simulink model "scara_2018a"  (R2018a)
settings: Solver=VariableStepAuto  StartTime=0.0  StopTime=inf  RelTol=1e-3
libraries: simulink x4, simulink_extras x2
settings Model: Creator=Bartlomiej Mroz  LastModifiedBy=Duch Kraftu
settings DebuggingCC: LibraryContextMissingDiagnostic=warning
settings SFSimCC: SimUseLocalCustomCode=on
settings RTWCC: RTWUseLocalCustomCode=on

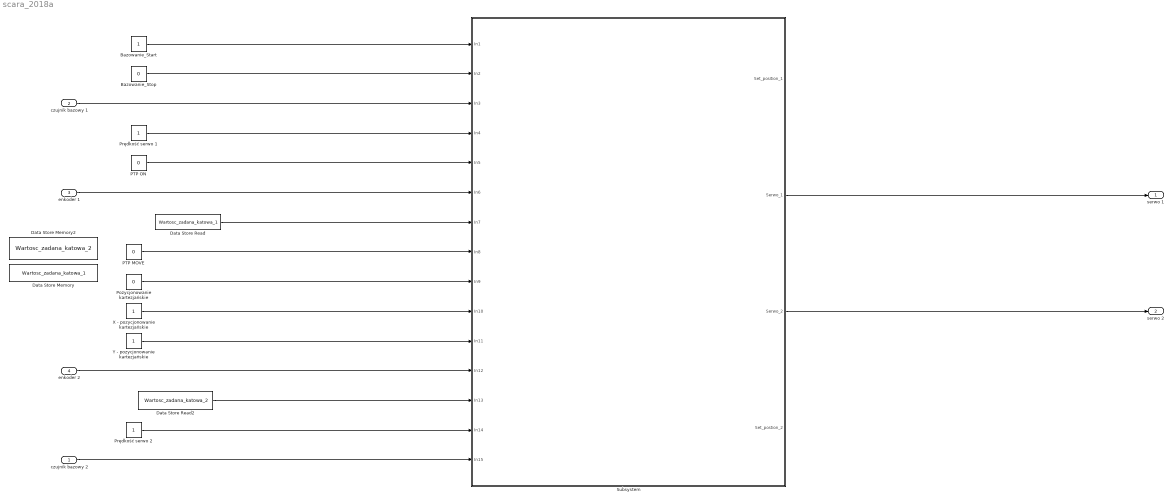
== system scara_2018a ==
  czujnik bazowy 2 : Inport
  czujnik bazowy 1 : Inport  Port=2
  enkoder 1 : Inport  Port=3
  enkoder 2 : Inport  Port=4
  " Bazowanie_Stop" : Constant  Value=0
  Bazowanie_Start : Constant
  Data Store Memory : DataStoreMemory  DataStoreName=Wartosc_zadana_katowa_1  ReadBeforeWriteMsg=warning  WriteAfterWriteMsg=warning  WriteAfterReadMsg=warning  ShowAdditionalParam=off
  Data Store Memory2 : DataStoreMemory  DataStoreName=Wartosc_zadana_katowa_2  ReadBeforeWriteMsg=warning  WriteAfterWriteMsg=warning  WriteAfterReadMsg=warning  ShowAdditionalParam=off
  Data Store Read : DataStoreRead  DataStoreName=Wartosc_zadana_katowa_1
  Data Store Read2 : DataStoreRead  DataStoreName=Wartosc_zadana_katowa_2
  PTP MOVE : Constant  Value=0
  "PTP ON " : Constant  Value=0
  "Pozycjonowanie kartezjańskie " : Constant  Value=0
  Prędkość serwo 1 : Constant
  Prędkość serwo 2 : Constant
  Subsystem : Subsystem
  X - pozycjonowanie kartezjańskie : Constant
  Y - pozycjonowanie kartezjańskie : Constant
  serwo 1 : Outport  VectorParamsAs1DForOutWhenUnconnected=on
  serwo 2 : Outport  Port=2  VectorParamsAs1DForOutWhenUnconnected=on
  wires:
  Bazowanie_Start/1 -> Subsystem/1(In1)
  " Bazowanie_Stop"/1 -> Subsystem/2(In2)
  czujnik bazowy 1/1 -> Subsystem/3(In3)
  Prędkość serwo 1/1 -> Subsystem/4(In4)
  "PTP ON "/1 -> Subsystem/5(In5)
  enkoder 1/1 -> Subsystem/6(In6)
  Data Store Read/1 -> Subsystem/7(In7)
  PTP MOVE/1 -> Subsystem/8(In8)
  "Pozycjonowanie kartezjańskie "/1 -> Subsystem/9(In9)
  X - pozycjonowanie kartezjańskie/1 -> Subsystem/10(In10)
  Y - pozycjonowanie kartezjańskie/1 -> Subsystem/11(In11)
  enkoder 2/1 -> Subsystem/12(In12)
  Data Store Read2/1 -> Subsystem/13(In13)
  Prędkość serwo 2/1 -> Subsystem/14(In14)
  czujnik bazowy 2/1 -> Subsystem/15(In15)
  Subsystem/2(Serwo_1) -> serwo 1/1
  Subsystem/3(Serwo_2) -> serwo 2/1

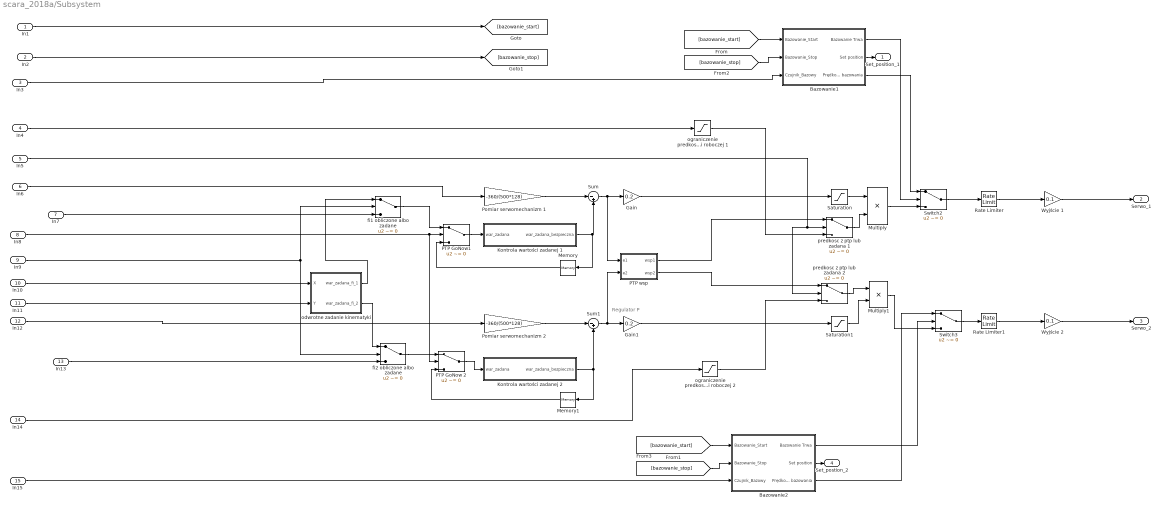
== system scara_2018a/Subsystem ==
  note: Regulator P
  In1 : Inport
  In2 : Inport  Port=2
  In3 : Inport  Port=3
  In4 : Inport  Port=4
  In5 : Inport  Port=5
  In6 : Inport  Port=6
  In7 : Inport  Port=7
  In8 : Inport  Port=8
  In9 : Inport  Port=9
  In10 : Inport  Port=10
  In11 : Inport  Port=11
  In12 : Inport  Port=12
  In13 : Inport  Port=13
  In14 : Inport  Port=14
  In15 : Inport  Port=15
  Bazowanie1 : Subsystem
  Bazowanie2 : Subsystem
  Gain : Gain  Gain=0.2
  Gain1 : Gain  Gain=0.2
  "Kontrola wartości zadanej 1 " : Subsystem
  Kontrola wartości zadanej 2 : Subsystem
  Memory : Memory
  Memory1 : Memory
  Multiply : Product
  Multiply1 : Product
  PTP GoNow 2 : Switch  Criteria=u2 ~= 0
  PTP GoNow1 : Switch  Criteria=u2 ~= 0
  "PTP wsp " : MATLAB Function  TreatAsAtomicUnit=on
  Pomiar serwomechanizm 1 : Gain  Gain=-360/(500*128)
  Pomiar serwomechanizm 2 : Gain  Gain=-360/(500*128)
  Rate Limiter : RateLimiter  RisingSlewLimit=50  FallingSlewLimit=-50  SampleTimeMode=inherited
  Rate Limiter1 : RateLimiter  RisingSlewLimit=50  FallingSlewLimit=-50  SampleTimeMode=inherited
  Saturation : Saturate  UpperLimit=3  LowerLimit=-3
  Saturation1 : Saturate  UpperLimit=3  LowerLimit=-3
  Sum : Sum  Inputs=|-+
  Sum1 : Sum  Inputs=|-+
  Switch2 : Switch  Criteria=u2 ~= 0
  Switch3 : Switch  Criteria=u2 ~= 0
  Wyjście 1 : Gain  Gain=0.1
  Wyjście 2 : Gain  Gain=0.1
  fi1 obliczone albo zadane : Switch  Criteria=u2 ~= 0
  fi2 obliczone albo zadane : Switch  Criteria=u2 ~= 0
  odwrotne zadanie kinematyki : Subsystem
  ograniczenie predkosci roboczej 1 : Saturate  UpperLimit=1  LowerLimit=0.05
  ograniczenie predkosci roboczej 2 : Saturate  UpperLimit=1  LowerLimit=0.05
  predkosc z ptp lub zadana 1 : Switch  Criteria=u2 ~= 0
  predkosc z ptp lub zadana 2 : Switch  Criteria=u2 ~= 0
  Set_position_1 : Outport  VectorParamsAs1DForOutWhenUnconnected=on
  Serwo_1 : Outport  Port=2  VectorParamsAs1DForOutWhenUnconnected=on
  Serwo_2 : Outport  Port=3  VectorParamsAs1DForOutWhenUnconnected=on
  Set_postion_2 : Outport  Port=4  VectorParamsAs1DForOutWhenUnconnected=on
  wires:
  In8/1 -> PTP GoNow 2/2, PTP GoNow1/2
  Bazowanie1/3(Prędkość bazowania) -> Switch2/1
  [bazowanie_start] -> Bazowanie1/1(Bazowanie_Start)
  Kontrola wartości zadanej 2/1(war_zadana_bezpieczna) -> Memory1/1, Sum1/2
  [bazowanie_stop] -> Bazowanie1/2("Bazowanie_Stop ")
  In9/1 -> fi1 obliczone albo zadane/2, fi2 obliczone albo zadane/2
  Bazowanie1/1("Bazowanie Trwa ") -> Switch2/2
  Multiply/1 -> Switch2/3
  Gain1/1 -> Saturation1/1
  [bazowanie_start] -> Bazowanie2/1(Bazowanie_Start)
  Sum/1 -> Gain/1, "PTP wsp "/1(e1)
  predkosc z ptp lub zadana 2/1 -> Multiply1/1
  [bazowanie_stop] -> Bazowanie2/2("Bazowanie_Stop ")
  In15/1 -> Bazowanie2/3(Czujnik_Bazowy)
  In12/1 -> Pomiar serwomechanizm 2/1
  ograniczenie predkosci roboczej 1/1 -> predkosc z ptp lub zadana 1/3
  Gain/1 -> Saturation/1
  ograniczenie predkosci roboczej 2/1 -> predkosc z ptp lub zadana 2/3
  In3/1 -> Bazowanie1/3(Czujnik_Bazowy)
  "Kontrola wartości zadanej 1 "/1(war_zadana_bezpieczna) -> Memory/1, Sum/2
  Bazowanie2/2("Set position ") -> Set_postion_2/1
  Sum1/1 -> Gain1/1, "PTP wsp "/2(e2)
  In5/1 -> predkosc z ptp lub zadana 2/2, predkosc z ptp lub zadana 1/2
  fi1 obliczone albo zadane/1 -> PTP GoNow1/1
  Saturation/1 -> Multiply/1
  Memory1/1 -> PTP GoNow 2/3
  Rate Limiter1/1 -> Wyjście 2/1
  Pomiar serwomechanizm 1/1 -> Sum/1
  Saturation1/1 -> Multiply1/2
  In6/1 -> Pomiar serwomechanizm 1/1
  In4/1 -> ograniczenie predkosci roboczej 1/1
  "PTP wsp "/2(wsp2) -> predkosc z ptp lub zadana 2/1
  Wyjście 1/1 -> Serwo_1/1
  In11/1 -> odwrotne zadanie kinematyki/2(Y)
  Pomiar serwomechanizm 2/1 -> Sum1/1
  fi2 obliczone albo zadane/1 -> PTP GoNow 2/1
  Wyjście 2/1 -> Serwo_2/1
  Bazowanie2/3(Prędkość bazowania) -> Switch3/1
  PTP GoNow 2/1 -> Kontrola wartości zadanej 2/1(war_zadana)
  odwrotne zadanie kinematyki/2(war_zadana_fi_2) -> fi2 obliczone albo zadane/1
  Switch3/1 -> Rate Limiter1/1
  Bazowanie2/1("Bazowanie Trwa ") -> Switch3/2
  PTP GoNow1/1 -> "Kontrola wartości zadanej 1 "/1(war_zadana)
  Memory/1 -> PTP GoNow1/3
  In14/1 -> ograniczenie predkosci roboczej 2/1
  predkosc z ptp lub zadana 1/1 -> Multiply/2
  Rate Limiter/1 -> Wyjście 1/1
  Switch2/1 -> Rate Limiter/1
  odwrotne zadanie kinematyki/1(war_zadana_fi_1) -> fi1 obliczone albo zadane/1
  In2/1 -> [bazowanie_stop]
  Multiply1/1 -> Switch3/3
  "PTP wsp "/1(wsp1) -> predkosc z ptp lub zadana 1/1
  In1/1 -> [bazowanie_start]
  In7/1 -> fi1 obliczone albo zadane/3
  Bazowanie1/2("Set position ") -> Set_position_1/1
  In13/1 -> fi2 obliczone albo zadane/3
  In10/1 -> odwrotne zadanie kinematyki/1(X)

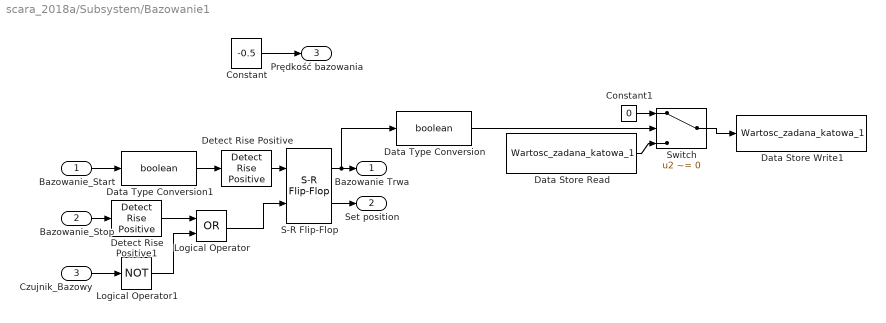
== system scara_2018a/Subsystem/Bazowanie1 ==
  Bazowanie_Start : Inport
  "Bazowanie_Stop " : Inport  Port=2
  Czujnik_Bazowy : Inport  Port=3
  Constant : Constant  Value=-0.5
  Constant1 : Constant  Value=0
  Data Store Read : DataStoreRead  DataStoreName=Wartosc_zadana_katowa_1
  Data Store Write1 : DataStoreWrite  DataStoreName=Wartosc_zadana_katowa_1
  Data Type Conversion : DataTypeConversion  OutDataTypeStr=boolean
  Data Type Conversion1 : DataTypeConversion  OutDataTypeStr=boolean
  Detect Rise Positive : simulink/Logic and Bit Operations/Detect Rise Positive  vinit=0  OutDataTypeStr=boolean
  Detect Rise Positive1 : simulink/Logic and Bit Operations/Detect Rise Positive  vinit=0  OutDataTypeStr=boolean
  Logical Operator : Logic  Operator=OR  AllPortsSameDT=off  OutDataTypeStr=boolean
  Logical Operator1 : Logic  Operator=NOT  AllPortsSameDT=off  OutDataTypeStr=boolean
  S-R Flip-Flop : simulink_extras/Flip Flops/S-R Flip-Flop  initial_condition=0
  Switch : Switch  Criteria=u2 ~= 0
  "Bazowanie Trwa " : Outport
  "Set position " : Outport  Port=2
  Prędkość bazowania : Outport  Port=3
  wires:
  "Bazowanie_Stop "/1 -> Detect Rise Positive1/1
  Czujnik_Bazowy/1 -> Logical Operator1/1
  Logical Operator1/1 -> Logical Operator/2
  Logical Operator/1 -> S-R Flip-Flop/2
  Bazowanie_Start/1 -> Data Type Conversion1/1
  S-R Flip-Flop/1 -> Data Type Conversion/1, "Bazowanie Trwa "/1
  S-R Flip-Flop/2 -> "Set position "/1
  Constant/1 -> Prędkość bazowania/1
  Switch/1 -> Data Store Write1/1
  Constant1/1 -> Switch/1
  Data Store Read/1 -> Switch/3
  Data Type Conversion/1 -> Switch/2
  Detect Rise Positive1/1 -> Logical Operator/1
  Data Type Conversion1/1 -> Detect Rise Positive/1
  Detect Rise Positive/1 -> S-R Flip-Flop/1

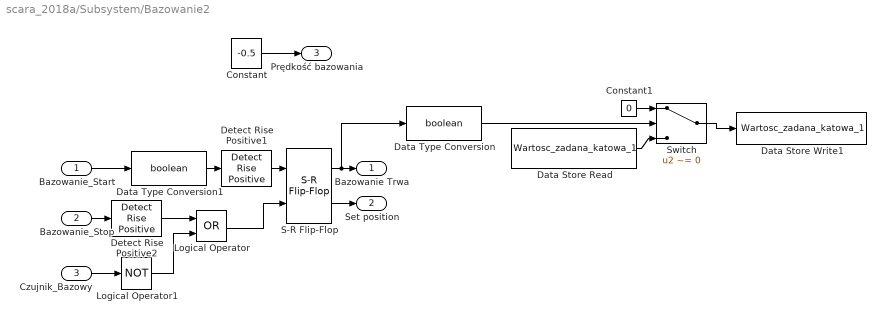
== system scara_2018a/Subsystem/Bazowanie2 ==
  Bazowanie_Start : Inport
  "Bazowanie_Stop " : Inport  Port=2
  Czujnik_Bazowy : Inport  Port=3
  Constant : Constant  Value=-0.5
  Constant1 : Constant  Value=0
  Data Store Read : DataStoreRead  DataStoreName=Wartosc_zadana_katowa_1
  Data Store Write1 : DataStoreWrite  DataStoreName=Wartosc_zadana_katowa_1
  Data Type Conversion : DataTypeConversion  OutDataTypeStr=boolean
  Data Type Conversion1 : DataTypeConversion  OutDataTypeStr=boolean
  Detect Rise Positive1 : simulink/Logic and Bit Operations/Detect Rise Positive  vinit=0  OutDataTypeStr=boolean
  Detect Rise Positive2 : simulink/Logic and Bit Operations/Detect Rise Positive  vinit=0  OutDataTypeStr=boolean
  Logical Operator : Logic  Operator=OR  AllPortsSameDT=off  OutDataTypeStr=boolean
  Logical Operator1 : Logic  Operator=NOT  AllPortsSameDT=off  OutDataTypeStr=boolean
  S-R Flip-Flop : simulink_extras/Flip Flops/S-R Flip-Flop  initial_condition=0
  Switch : Switch  Criteria=u2 ~= 0
  "Bazowanie Trwa " : Outport
  "Set position " : Outport  Port=2
  Prędkość bazowania : Outport  Port=3
  wires:
  "Bazowanie_Stop "/1 -> Detect Rise Positive2/1
  Czujnik_Bazowy/1 -> Logical Operator1/1
  Logical Operator1/1 -> Logical Operator/2
  Logical Operator/1 -> S-R Flip-Flop/2
  Bazowanie_Start/1 -> Data Type Conversion1/1
  S-R Flip-Flop/2 -> "Set position "/1
  Constant/1 -> Prędkość bazowania/1
  Data Store Read/1 -> Switch/3
  Switch/1 -> Data Store Write1/1
  Constant1/1 -> Switch/1
  S-R Flip-Flop/1 -> Data Type Conversion/1, "Bazowanie Trwa "/1
  Data Type Conversion/1 -> Switch/2
  Data Type Conversion1/1 -> Detect Rise Positive1/1
  Detect Rise Positive1/1 -> S-R Flip-Flop/1
  Detect Rise Positive2/1 -> Logical Operator/1

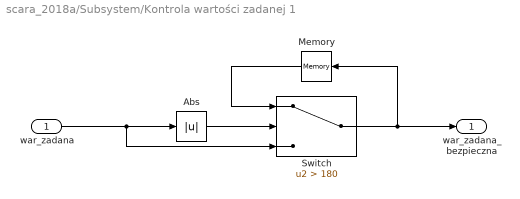
== system scara_2018a/Subsystem/Kontrola wartości zadanej 1  ==
  war_zadana : Inport
  Abs : Abs
  Memory : Memory
  Switch : Switch  Criteria=u2 > Threshold  Threshold=180
  war_zadana_bezpieczna : Outport
  wires:
  war_zadana/1 -> Switch/3, Abs/1
  Abs/1 -> Switch/2
  Switch/1 -> Memory/1, war_zadana_bezpieczna/1
  Memory/1 -> Switch/1

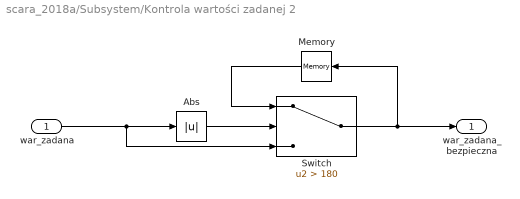
== system scara_2018a/Subsystem/Kontrola wartości zadanej 2 ==
  war_zadana : Inport
  Abs : Abs
  Memory : Memory
  Switch : Switch  Criteria=u2 > Threshold  Threshold=180
  war_zadana_bezpieczna : Outport
  wires:
  Memory/1 -> Switch/1
  Switch/1 -> war_zadana_bezpieczna/1, Memory/1
  Abs/1 -> Switch/2
  war_zadana/1 -> Abs/1, Switch/3

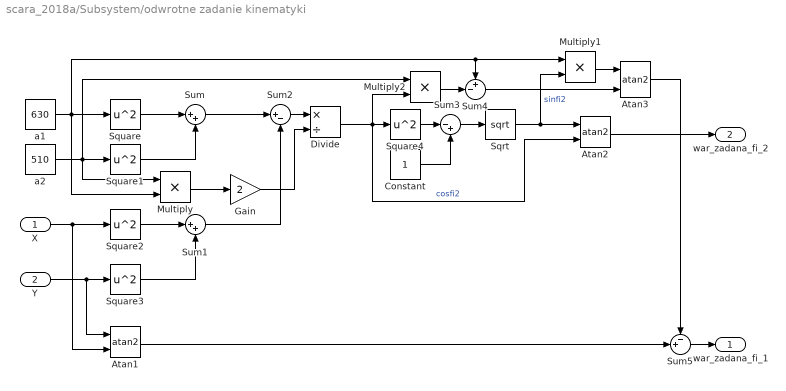
== system scara_2018a/Subsystem/odwrotne zadanie kinematyki ==
  X : Inport
  Y : Inport  Port=2
  Atan1 : Trigonometry  Operator=atan2
  Atan2 : Trigonometry  Operator=atan2
  Atan3 : Trigonometry  Operator=atan2
  Constant : Constant
  Divide : Product  Inputs=*/
  Gain : Gain  Gain=2
  Multiply : Product
  Multiply1 : Product
  Multiply2 : Product
  Sqrt : Sqrt  SaturateOnIntegerOverflow=on
  Square{,1..4} (5 alike) : Math  Operator=square  SaturateOnIntegerOverflow=on
  Sum : Sum  Inputs=|++
  Sum1 : Sum  Inputs=|++
  Sum2 : Sum  Inputs=|+-
  Sum3 : Sum  Inputs=|-+
  Sum4 : Sum  Inputs=+-|
  Sum5 : Sum  Inputs=-+|
  a1 : Constant  Value=630
  a2 : Constant  Value=510
  war_zadana_fi_1 : Outport
  war_zadana_fi_2 : Outport  Port=2
  wires:
  a2/1 -> Multiply2/1, Square1/1, Multiply/1
  X/1 -> Atan1/2, Square2/1
  Y/1 -> Atan1/1, Square3/1
  Multiply/1 -> Gain/1
  Square/1 -> Sum/1
  Square1/1 -> Sum/2
  Square2/1 -> Sum1/1
  Square3/1 -> Sum1/2
  Sum/1 -> Sum2/1
  Sum1/1 -> Sum2/2
  Sum2/1 -> Divide/1
  Gain/1 -> Divide/2
  Divide/1 -> Multiply2/2, Atan2/2, Square4/1  "cosfi2"
  Square4/1 -> Sum3/1
  Sum3/1 -> Sqrt/1
  Constant/1 -> Sum3/2
  Sqrt/1 -> Multiply1/2, Atan2/1  "sinfi2"
  Atan2/1 -> war_zadana_fi_2/1
  a1/1 -> Sum4/1, Multiply1/1, Square/1, Multiply/2
  Multiply2/1 -> Sum4/2
  Multiply1/1 -> Atan3/1
  Sum4/1 -> Atan3/2
  Sum5/1 -> war_zadana_fi_1/1
  Atan1/1 -> Sum5/2
  Atan3/1 -> Sum5/1

== matlab function scara_2018a/Subsystem/PTP wsp  ==
  data: e1 input; wsp1 output; e2 input; wsp2 output
function [wsp1,wsp2] = fcn(e1,e2)
denum = max(e1,e2);
wsp1 = e1/denum;
wsp2 = e2/denum;
